simulink model "Wind_Turbine"  (R2023b)
settings: Solver=VariableStepAuto  StartTime=0.0  StopTime=10.0  RelTol=1e-3  AbsTol=1e-3
settings Model: Creator=3.22  LastModifiedBy=3.22
settings SolverCC: AutoScaleAbsTol=off  AlgebraicLoopSolver=TrustRegion  MaxZcPerStep=1
settings DebuggingCC: UnconnectedInputMsg=warning  UnconnectedOutputMsg=warning  UnconnectedLineMsg=warning  SymbolicDimsDataTypeCodeGenerationDiagnostic=none
settings ModelReferenceCC: EnableRefExpFcnMdlSchedulingChecks=on
settings SFSimCC: CustomCodeUndefinedFunction=UseInterfaceOnly
settings RTWCC: DLArmComputeVersion=19.05
settings SimscapeCC: SimscapeLogType=all  SimscapeLogSimulationStatistics=on  SimscapeLogDataHistory=10000

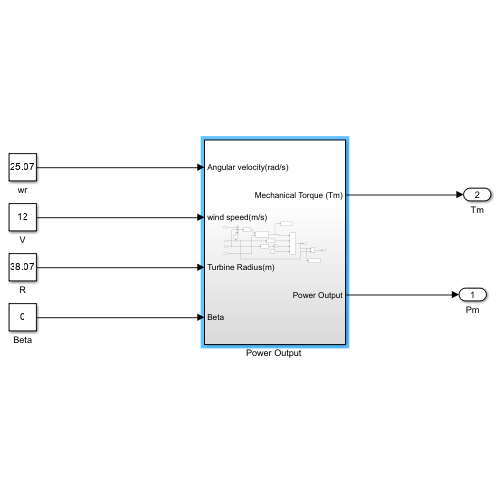
[thumbnail: Simulink's stored preview of the top-level diagram]
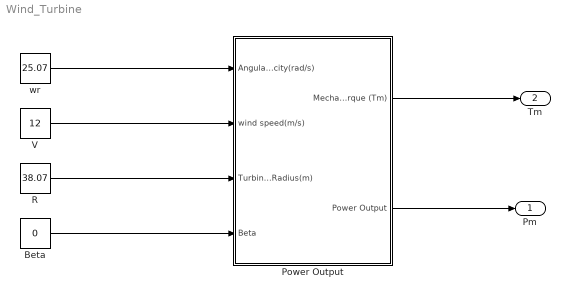
== system Wind_Turbine ==
  Beta : Constant  Value=0
  "Power Output " : Subsystem
  R : Constant  Value=38.07
  V : Constant  Value=12
  wr : Constant  Value=25.07
  Pm : Outport
  Tm : Outport  Port=2
  wires:
  "Power Output "/2(Power Output) -> Pm/1
  wr/1 -> "Power Output "/1(Angular velocity(rad/s))
  V/1 -> "Power Output "/2(wind speed(m/s))
  R/1 -> "Power Output "/3("Turbine Radius(m) ")
  "Power Output "/1(Mechanical Torque (Tm)) -> Tm/1
  Beta/1 -> "Power Output "/4(Beta)

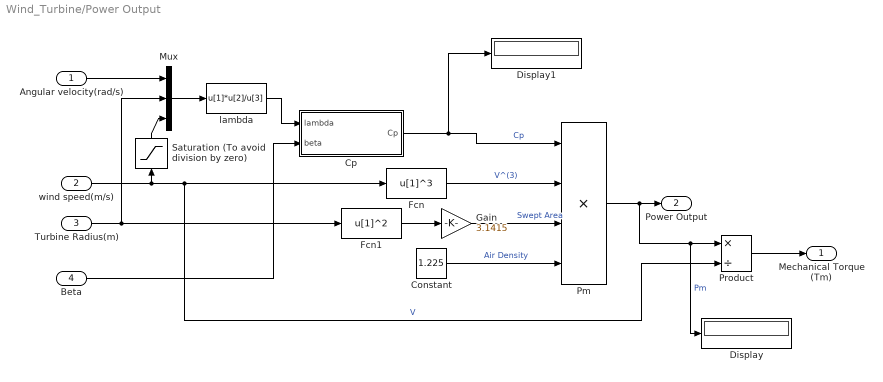
== system Wind_Turbine/Power Output  ==
  Angular velocity(rad/s) : Inport
  wind speed(m/s) : Inport  Port=2
  "Turbine Radius(m) " : Inport  Port=3
  Beta : Inport  Port=4
  Constant : Constant  Value=1.225
  Cp : Subsystem
  Display : Display
  Display1 : Display
  Fcn : Fcn  Expr=u[1]^3
  Fcn1 : Fcn  Expr=u[1]^2
  Gain : Gain  Gain=3.1415
  Mux : Mux  Inputs=3
  Pm : Product  Inputs=4
  Product : Product  Inputs=*/
  Saturation (To avoid division by zero) : Saturate  UpperLimit=1e6  LowerLimit=1e-6
  lambda : Fcn  Expr=u[1]*u[2]/u[3]
  Mechanical Torque (Tm) : Outport
  Power Output : Outport  Port=2
  wires:
  Cp/1(Cp) -> Display1/1, Pm/1  "Cp"
  Pm/1 -> Power Output/1, Display/1, Product/1  "Pm"
  wind speed(m/s)/1 -> Saturation (To avoid division by zero)/1, Product/2, Fcn/1  "V"
  Fcn/1 -> Pm/2  "V^(3)"
  Fcn1/1 -> Gain/1
  "Turbine Radius(m) "/1 -> Fcn1/1, Mux/2
  Gain/1 -> Pm/3  "Swept Area"
  Constant/1 -> Pm/4  "Air Density"
  Angular velocity(rad/s)/1 -> Mux/1
  lambda/1 -> Cp/1(lambda)
  Mux/1 -> lambda/1
  Saturation (To avoid division by zero)/1 -> Mux/3
  Product/1 -> Mechanical Torque (Tm)/1
  Beta/1 -> Cp/2(beta)

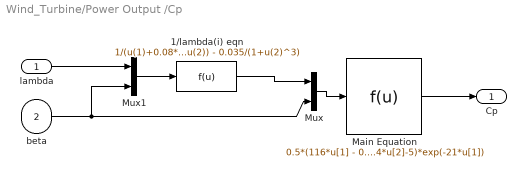
== system Wind_Turbine/Power Output /Cp ==
  lambda : Inport
  beta : Inport  Port=2
  1/lambda(i) eqn : Fcn  Expr=1/(u(1)+0.08*u(2)) - 0.035/(1+u(2)^3)
  Main Equation : Fcn  Expr=0.5*(116*u[1] - 0.4*u[2]-5)*exp(-21*u[1])
  Mux : Mux  Inputs=2
  Mux1 : Mux  Inputs=2
  Cp : Outport
  wires:
  Mux/1 -> Main Equation/1
  1/lambda(i) eqn/1 -> Mux/1
  beta/1 -> Mux1/2, Mux/2
  lambda/1 -> Mux1/1
  Mux1/1 -> 1/lambda(i) eqn/1
  Main Equation/1 -> Cp/1
